simulink library "Kitchen_Lib"  (R2023a)
settings: Solver=VariableStepAuto  StartTime=0.0  StopTime=10.0  RelTol=1e-3  EnableMultiTasking=on
undefined symbols (not defined in the file): Kitc_BusTyp_P, Kitc_BusTypSkyr_C, Kitc_ColrLedColrls_C, Kitc_ColrLedGrn_C, Kitc_ColrLedRed_C, Kitc_ColrLedYlw_C, Kitc_StDgnWtrTank_C, Kitc_StElecPlugScktOffByClmp50_P, Kitc_StsDlyBlink_C, Kitc_StsErrBlink_C, Kitc_StsFctAcvn_P, Kitc_StsInfoBlink_C, Kitc_StsKitchnOffAutoIgOff_P, Kitc_StsKitchnOffBySwt_P, Kitc_StsKitchnOffDoorLockd_P, Kitc_StsKitchnOffIgOff_P, Kitc_StsKitchnOffUv_P, Kitc_StsKitchnOnBySwt_P, Kitc_StsKitchnOnNVM_P, Kitc_StsLedOff_C, Kitc_StsLedOn_C, Kitc_StsLrgCnsAcv_P, Kitc_StTrfrAnSwtInstd_P, Kitc_StTrfrSwtInstd_P, Kitc_TiKitcRefgtrOffDly_P, Kitc_ULowrThdBat_C, Kitc_UUpprThdBat_C, Kitc_ValFalse_C, Kitc_ValPwmFreq2_C, Kitc_ValPwmFreq_C, Kitc_ValTrue_C
libraries: MAN_Library x50, E2E_Lib x3
(part 3 of 13)

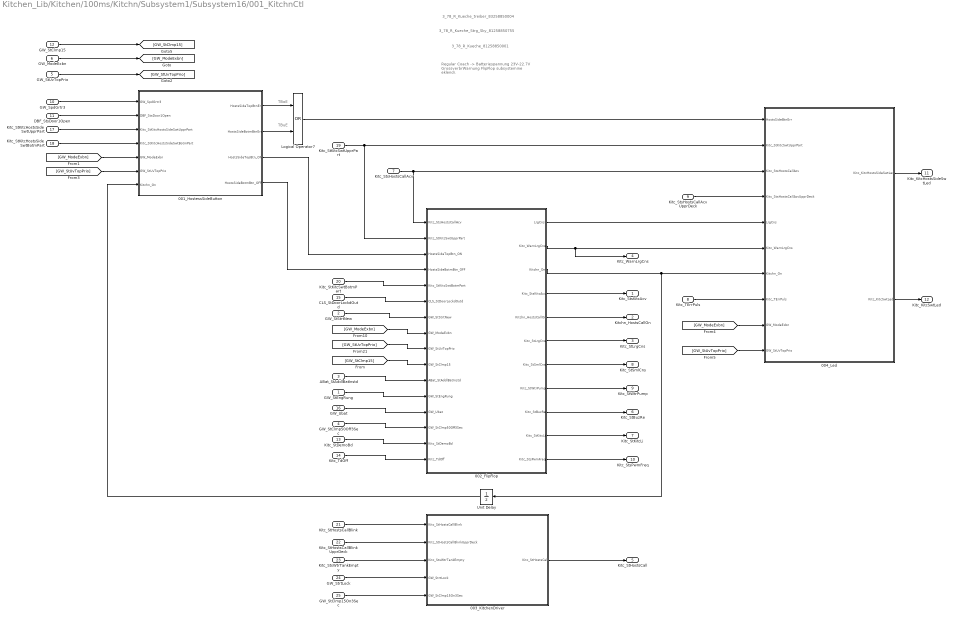
== system Kitchen_Lib/Kitchen/100ms/Kitchn/Subsystem1/Subsystem16/001_KitchnCtl ==
  note: 3_78_R_Kueche_treiber_83258850004
  note: Regular Coach -> Batteriespannung 23V-22.7V
      | GrossverbrWarnung
      |
      | FlipFlop subsystemine eklendi.
  note: 3_78_R_Kueche_81258850001
  note: TBuE
  note: TBoE
  note: 3_78_R_Kueche_Strg_Sky_81258850755
  GW_StEngRung : Inport
  "GW_StStrtNew " : Inport  Port=2
  ABat_StAddlBatInstd : Inport  Port=3
  "GW_StClmp50Off3Sec " : Inport  Port=4
  "GW_StUvTopPrio " : Inport  Port=5
  "GW_ModeExbn " : Inport  Port=6
  Kitc_StsHostsCallAcv : Inport  Port=7
  Kitc_TErrPuls : Inport  Port=8
  Kitc_StsHostsCallAcvUpprDeck : Inport  Port=9
  GW_SpdGrtr3 : Inport  Port=10
  DBF_StsDoor1Open : Inport  Port=11
  GW_StClmp15 : Inport  Port=12
  Kitc_StDemoBd : Inport  Port=13
  Kitc_TdOff : Inport  Port=14
  CLS_StDoorLockdOutd : Inport  Port=15
  "GW_Ubat " : Inport  Port=16
  Kitc_StKitcHostsSideSwtUpprPart : Inport  Port=17
  Kitc_StKitcHostsSideSwtBotmPart : Inport  Port=18
  Kitc_StKitcSwtUpprPart : Inport  Port=19
  Kitc_StKitcSwtBotmPart : Inport  Port=20
  Kitc_StHostsCallBlink : Inport  Port=21
  Kitc_StHostsCallBlinkUpprDeck : Inport  Port=22
  Kitc_StsWtrTankEmpty : Inport  Port=23
  "GW_StrtLock " : Inport  Port=24
  "GW_StClmp15On3Sec " : Inport  Port=25
  001_HostessSideButton : Subsystem
  002_FlipFlop : Subsystem
  003_KitchenDriver : Subsystem
  004_Led : Subsystem
  Logical Operator7 : Logic  Operator=OR  AllPortsSameDT=off  OutDataTypeStr=boolean
  Unit Delay : UnitDelay  SampleTime=-1  HasFrameUpgradeWarning=on
  Kitc_StsKitcAcv : Outport
  Kitchn_HostsCallOn : Outport  Port=2
  Kitc_StLrgCns : Outport  Port=3
  Kitc_WarnLrgCns : Outport  Port=4
  Kitc_StHostsCall : Outport  Port=5
  Kitc_StBuzRe : Outport  Port=6
  Kitc_StKitcLi : Outport  Port=7
  Kitc_StSmlCns : Outport  Port=8
  Kitc_StWtrPump : Outport  Port=9
  Kitc_StsPwmFreq : Outport  Port=10
  Kitc_KitcHostsSideSwtLed : Outport  Port=11
  Kitc_KitcSwtLed : Outport  Port=12
  wires:
  Kitc_StKitcSwtUpprPart/1 -> 002_FlipFlop/2(Kitc_StKitcSwtUpprPart), 004_Led/2(Kitc_StKitcSwtUpprPart)
  "GW_ModeExbn "/1 -> [GW_ModeExbn]
  "GW_StUvTopPrio "/1 -> [GW_StUvTopPrio]
  Kitc_StDemoBd/1 -> 002_FlipFlop/15(Kitc_StDemoBd)
  Kitc_TdOff/1 -> 002_FlipFlop/16(Kitc_TdOff)
  GW_StClmp15/1 -> [GW_StClmp15]
  Kitc_StsHostsCallAcv/1 -> 002_FlipFlop/1(Kitc_StsHostsCallAcv), 004_Led/3(Kitc_StsHostsCallAcv)
  Kitc_StsHostsCallAcvUpprDeck/1 -> 004_Led/4(Kitc_StsHostsCallAcvUpprDeck)
  Logical Operator7/1 -> 004_Led/1(HostsSideBtnErr)
  002_FlipFlop/3(Kitchn_On) -> 004_Led/7(Kitchn_On), Unit Delay/1
  Kitc_StKitcSwtBotmPart/1 -> 002_FlipFlop/5(Kitc_StKitcSwtBotmPart)
  CLS_StDoorLockdOutd/1 -> 002_FlipFlop/6(CLS_StDoorLockdOutd)
  [GW_StUvTopPrio] -> 002_FlipFlop/9("GW_StUvTopPrio ")
  [GW_ModeExbn] -> 002_FlipFlop/8("GW_ModeExbn ")
  "GW_StStrtNew "/1 -> 002_FlipFlop/7("GW_StStrtNew ")
  002_FlipFlop/4(Kitc_StsKitcAcv) -> Kitc_StsKitcAcv/1
  002_FlipFlop/5(Kitchn_HostsCallOn) -> Kitchn_HostsCallOn/1
  002_FlipFlop/6(Kitc_StLrgCns) -> Kitc_StLrgCns/1
  ABat_StAddlBatInstd/1 -> 002_FlipFlop/11(ABat_StAddlBatInstd)
  GW_StEngRung/1 -> 002_FlipFlop/12(GW_StEngRung)
  002_FlipFlop/2(Kitc_WarnLrgCns) -> Kitc_WarnLrgCns/1, 004_Led/6(Kitc_WarnLrgCns)
  "GW_StClmp50Off3Sec "/1 -> 002_FlipFlop/14("GW_StClmp50Off3Sec ")
  "GW_Ubat "/1 -> 002_FlipFlop/13("GW_Ubat ")
  002_FlipFlop/1(LrgCns) -> 004_Led/5(LrgCns)
  GW_SpdGrtr3/1 -> 001_HostessSideButton/1(GW_SpdGrtr3)
  DBF_StsDoor1Open/1 -> 001_HostessSideButton/2(DBF_StsDoor1Open)
  Kitc_StKitcHostsSideSwtUpprPart/1 -> 001_HostessSideButton/3(Kitc_StKitcHostsSideSwtUpprPart)
  Kitc_StKitcHostsSideSwtBotmPart/1 -> 001_HostessSideButton/4(Kitc_StKitcHostsSideSwtBotmPart)
  001_HostessSideButton/1(HostsSideTopBtnErr) -> Logical Operator7/1
  001_HostessSideButton/2(HostsSideBotmBtnErr) -> Logical Operator7/2
  001_HostessSideButton/3(HostsSideTopBtn_ON) -> 002_FlipFlop/3(HostsSideTopBtn_ON)
  001_HostessSideButton/4(HostsSideBotmBtn_OFF) -> 002_FlipFlop/4(HostsSideBotmBtn_OFF)
  Kitc_StsWtrTankEmpty/1 -> 003_KitchenDriver/3(Kitc_StsWtrTankEmpty)
  Kitc_StHostsCallBlink/1 -> 003_KitchenDriver/1(Kitc_StHostsCallBlink)
  "GW_StClmp15On3Sec "/1 -> 003_KitchenDriver/5("GW_StClmp15On3Sec ")
  003_KitchenDriver/1(Kitc_StHostsCall) -> Kitc_StHostsCall/1
  "GW_StrtLock "/1 -> 003_KitchenDriver/4("GW_StrtLock ")
  Kitc_StHostsCallBlinkUpprDeck/1 -> 003_KitchenDriver/2(Kitc_StHostsCallBlinkUpprDeck)
  [GW_ModeExbn] -> 001_HostessSideButton/5("GW_ModeExbn ")
  Unit Delay/1 -> 001_HostessSideButton/7(Kitchn_On)
  Kitc_TErrPuls/1 -> 004_Led/8(Kitc_TErrPuls)
  002_FlipFlop/7(Kitc_StSmlCns) -> Kitc_StSmlCns/1
  002_FlipFlop/8(Kitc_StWtrPump) -> Kitc_StWtrPump/1
  002_FlipFlop/9(Kitc_StBuzRe) -> Kitc_StBuzRe/1
  [GW_StUvTopPrio] -> 001_HostessSideButton/6("GW_StUvTopPrio ")
  [GW_ModeExbn] -> 004_Led/9("GW_ModeExbn ")
  [GW_StUvTopPrio] -> 004_Led/10("GW_StUvTopPrio ")
  002_FlipFlop/10(Kitc_StKitcLi) -> Kitc_StKitcLi/1
  [GW_StClmp15] -> 002_FlipFlop/10(GW_StClmp15)
  002_FlipFlop/11(Kitc_StsPwmFreq) -> Kitc_StsPwmFreq/1
  004_Led/1(Kitc_KitcHostsSideSwtLed) -> Kitc_KitcHostsSideSwtLed/1
  004_Led/2(Kitc_KitcSwtLed) -> Kitc_KitcSwtLed/1

== system Kitchen_Lib/Kitchen/100ms/Kitchn/Subsystem1/Subsystem16/002_ElectPlgSckt ==
  note: O_368_Steckdose_mit_KL50_aus_33258850303
  note: Parameter Kueche_Steckd_Aus_Kl50_P is deleted
  "GW_StrtClmp50 " : Inport
  Constant1 : Constant  Value=Kitc_StElecPlugScktOffByClmp50_P
  Constant2 : Constant  Value=Kitc_ValFalse_C
  Logical Operator : Logic  Operator=NOT  AllPortsSameDT=off  OutDataTypeStr=boolean
  Logical Operator1 : Logic  AllPortsSameDT=off  OutDataTypeStr=boolean
  Multiport Switch : MultiPortSwitch  DataPortOrder=Zero-based contiguous  Inputs=2  zeroidx=on  SaturateOnIntegerOverflow=off  InputSameDT=off
  Kitc_StElecPlgSckt : Outport
  wires:
  Multiport Switch/1 -> Kitc_StElecPlgSckt/1
  Constant2/1 -> Multiport Switch/1
  "GW_StrtClmp50 "/1 -> Logical Operator1/1
  Logical Operator/1 -> Multiport Switch/2
  Logical Operator1/1 -> Multiport Switch/3, Logical Operator/1
  Constant1/1 -> Logical Operator1/2

== system Kitchen_Lib/Kitchen/100ms/Kitchn/Subsystem1/Subsystem16/003_Refgtr ==
  note: O_368_Kuehlschrank_33258850044
  note: 3_78_R_Kuehlschrank_vorne _81258850186
  note: Parameter
      | Kueche_Kuehlbox_nur_bei_KL15_P
      | is deleted
  note: Parameter
      | Kueche_Kuehlbox_nur_bei_Motorlauf_P
      | is deleted
  GW_StClmp15 : Inport
  "GW_StEngAcv " : Inport  Port=2
  GW_StClmpRdo : Inport  Port=3
  "GW_StUvLoPrio " : Inport  Port=4
  "GW_StUvTopPrio " : Inport  Port=5
  Constant : Constant  Value=Kitc_TiKitcRefgtrOffDly_P
  Constant2 : Constant  Value=Kitc_ValFalse_C
  Constant3 : Constant  Value=Kitc_ValFalse_C
  Data Store Read : DataStoreRead  DataStoreName=Kitc_TiKitcRefgtrOffDlyNv  IndexOptions=Index vector (dialog)  Indices=1  OutputSizes=1
  Data Type Conversion : DataTypeConversion  OutDataTypeStr=uint32  SaturateOnIntegerOverflow=off  RndMeth=Floor
  Data Type Conversion1 : DataTypeConversion  OutDataTypeStr=boolean  SaturateOnIntegerOverflow=off  RndMeth=Floor
  Logical Operator{,3,7..8} (4 alike) : Logic  Operator=NOT  AllPortsSameDT=off  OutDataTypeStr=boolean
  Logical Operator{1,4,6,9} (4 alike) : Logic  AllPortsSameDT=off  OutDataTypeStr=boolean
  Logical Operator2 : Logic  Inputs=3  AllPortsSameDT=off  OutDataTypeStr=boolean
  Logical Operator5 : Logic  Operator=OR  Inputs=3  AllPortsSameDT=off  OutDataTypeStr=boolean
  Switch : Switch  Criteria=u2 ~= 0  SaturateOnIntegerOverflow=off  InputSameDT=off
  Terminator4 : Terminator
  TurnOffDelay : MAN_Library/TurnOffDelay  CycleTime=Cycle Time: 10 Ms
  Kitc_StRefgtr : Outport
  "Kitc_StFrntRefgtr " : Outport  Port=2
  wires:
  Data Type Conversion1/1 -> Switch/2
  Constant/1 -> Switch/3
  Data Store Read/1 -> Switch/1, Data Type Conversion1/1
  Switch/1 -> Data Type Conversion/1
  Constant2/1 -> Logical Operator1/2, Logical Operator/1
  Logical Operator/1 -> Logical Operator2/1
  GW_StClmpRdo/1 -> Logical Operator2/2
  Constant3/1 -> Logical Operator4/1, Logical Operator3/1
  Logical Operator3/1 -> Logical Operator2/3
  "GW_StEngAcv "/1 -> Logical Operator4/2
  Logical Operator2/1 -> Logical Operator5/2
  Logical Operator1/1 -> Logical Operator5/1
  Logical Operator4/1 -> Logical Operator5/3
  Logical Operator5/1 -> TurnOffDelay/1
  TurnOffDelay/1 -> Logical Operator6/1
  Logical Operator6/1 -> Kitc_StRefgtr/1
  "GW_StUvLoPrio "/1 -> Logical Operator7/1
  Logical Operator7/1 -> Logical Operator6/2
  "GW_StUvTopPrio "/1 -> Logical Operator8/1
  Logical Operator8/1 -> Logical Operator9/1
  Logical Operator9/1 -> "Kitc_StFrntRefgtr "/1
  GW_StClmp15/1 -> Logical Operator1/1, Logical Operator9/2
  Data Type Conversion/1 -> TurnOffDelay/2
  TurnOffDelay/2 -> Terminator4/1

== system Kitchen_Lib/Kitchen/100ms/Kitchn/Subsystem1/Subsystem16/004_Trfr ==
  note: 3_78_R_Umformer_81258850049
  "Kitc_StTrfrSwt " : Inport
  GW_StClmp15 : Inport  Port=2
  "GW_StUvNormPrio " : Inport  Port=3
  Kitc_StTrfrSwtUpprPart : Inport  Port=4
  Kitc_StTrfrSwtTopBtn : Inport  Port=5
  Kitc_StTrfrSwtLowrPart : Inport  Port=6
  Kitc_StTrfrBotmBtm : Inport  Port=7
  Kitc_StTrfrWoutNewStrt : Inport  Port=8
  "GW_StClmp50Off3Sec " : Inport  Port=9
  ABat_StAddlBatInstd : Inport  Port=10
  "GW_StStrtNew " : Inport  Port=11
  GW_StEngRung : Inport  Port=12
  Kitc_StsKitcAcv : Inport  Port=13
  001_AutomaticControlKitchenRelease : Subsystem
  002_FlipFlop : Subsystem
  003_TrfrSwtLed : Subsystem
  Constant13 : Constant  Value=Kitc_StTrfrSwtInstd_P
  Constant2 : Constant  Value=Kitc_ValTrue_C
  Constant3 : Constant  Value=Kitc_StTrfrAnSwtInstd_P
  Ground : Ground
  Ground1 : Ground
  LEDSignal_Subsytem : E2E_Lib/LEDSignal_Subsytem
  Logical Operator1 : Logic  Operator=OR  Inputs=3  AllPortsSameDT=off  OutDataTypeStr=boolean
  Logical Operator2 : Logic  AllPortsSameDT=off  OutDataTypeStr=boolean
  Logical Operator5 : Logic  Operator=NOT  AllPortsSameDT=off  OutDataTypeStr=boolean
  Multiport Switch : MultiPortSwitch  DataPortOrder=Zero-based contiguous  Inputs=2  zeroidx=on  SaturateOnIntegerOverflow=off  InputSameDT=off
  PushPull : Subsystem
  Kitc_StTrfrInstd : Outport
  Kitc_StTrfrHiSide : Outport  Port=2
  Kitc_StTrfrLoSide : Outport  Port=3
  Kitc_TrfrSwtLed : Outport  Port=4
  wires:
  "Kitc_StTrfrSwt "/1 -> Logical Operator1/1
  Constant13/1 -> Logical Operator1/2
  Multiport Switch/1 -> Logical Operator2/2
  "GW_StClmp50Off3Sec "/1 -> Logical Operator5/1
  Logical Operator2/1 -> PushPull/1(In1)
  PushPull/1(HS) -> Kitc_StTrfrHiSide/1
  PushPull/2(LS) -> Kitc_StTrfrLoSide/1
  Constant2/1 -> Kitc_StTrfrInstd/1
  Logical Operator1/1 -> Multiport Switch/1, 002_FlipFlop/1(TrfrSwt)
  002_FlipFlop/1(Fnc_On) -> Multiport Switch/3, 003_TrfrSwtLed/1(Fnc_On)
  Kitc_StTrfrSwtUpprPart/1 -> 002_FlipFlop/2(Kitc_StTrfrSwtUpprPart)
  Kitc_StTrfrSwtTopBtn/1 -> 002_FlipFlop/3(Kitc_StTrfrSwtTopBtn)
  Kitc_StTrfrSwtLowrPart/1 -> 002_FlipFlop/4(Kitc_StTrfrSwtLowrPart)
  Kitc_StTrfrBotmBtm/1 -> 002_FlipFlop/5(Kitc_StTrfrBotmBtm)
  "GW_StStrtNew "/1 -> 002_FlipFlop/6("GW_StStrtNew ")
  Kitc_StTrfrWoutNewStrt/1 -> 002_FlipFlop/7(Kitc_StTrfrWoutNewStrt)
  [GW_StEngRung] -> 002_FlipFlop/8(GW_StEngRung)
  [ABat_StAddlBatInstd] -> 002_FlipFlop/9(ABat_StAddlBatInstd)
  [GW_StClmp15] -> 002_FlipFlop/10(GW_StClmp15)
  [GW_StUvNormPrio] -> 002_FlipFlop/11("GW_StUvNormPrio ")
  Logical Operator5/1 -> Logical Operator2/1
  GW_StClmp15/1 -> [GW_StClmp15], 001_AutomaticControlKitchenRelease/1(GW_StClmp15)
  "GW_StUvNormPrio "/1 -> [GW_StUvNormPrio], 001_AutomaticControlKitchenRelease/2("GW_StUvNormPrio ")
  ABat_StAddlBatInstd/1 -> [ABat_StAddlBatInstd], 001_AutomaticControlKitchenRelease/3(ABat_StAddlBatInstd)
  GW_StEngRung/1 -> 001_AutomaticControlKitchenRelease/4(GW_StEngRung), [GW_StEngRung]
  Kitc_StsKitcAcv/1 -> 001_AutomaticControlKitchenRelease/5(Kitc_StsKitcAcv)
  001_AutomaticControlKitchenRelease/1(Kitchen) -> Multiport Switch/2
  Constant3/1 -> Logical Operator1/3
  003_TrfrSwtLed/1(Kitc_ColrTrfrSwtLed) -> LEDSignal_Subsytem/1
  003_TrfrSwtLed/2(Kitc_StsTrfrSwtLed) -> LEDSignal_Subsytem/2
  Ground/1 -> LEDSignal_Subsytem/3
  Ground1/1 -> LEDSignal_Subsytem/4
  LEDSignal_Subsytem/1 -> Kitc_TrfrSwtLed/1

== system Kitchen_Lib/Kitchen/100ms/Kitchn/Subsystem1/Subsystem17/UINT32_Signal ==
  UINT32_SignalIn : Inport
  Constant : Constant  Value=uint32(0)
  Constant1 : Constant  Value=uint32(1)
  Constant2 : Constant  Value=uint32(4294967294)
  Constant3 : Constant  Value=uint32(4294967295)
  Data Type Conversion : DataTypeConversion  OutDataTypeStr=uint32  SaturateOnIntegerOverflow=off  RndMeth=Floor
  Relational Operator{,1..3} (4 alike) : RelationalOperator  Operator===  OutDataTypeStr=boolean  InputSameDT=off
  Terminator : Terminator
  Terminator1 : Terminator
  Error : Outport
  NotInstalled_NotAvailable : Outport  Port=2
  wires:
  Relational Operator3/1 -> NotInstalled_NotAvailable/1
  Relational Operator2/1 -> Error/1
  Data Type Conversion/1 -> Relational Operator/1, Relational Operator1/1, Relational Operator2/1, Relational Operator3/1
  Constant/1 -> Relational Operator/2
  UINT32_SignalIn/1 -> Data Type Conversion/1
  Constant3/1 -> Relational Operator3/2
  Constant1/1 -> Relational Operator1/2
  Relational Operator/1 -> Terminator/1
  Relational Operator1/1 -> Terminator1/1
  Constant2/1 -> Relational Operator2/2

== system Kitchen_Lib/Kitchen/100ms/Kitchn/Subsystem1/Subsystem19/003_TrfrSwtLed ==
  Fnc_On : Inport
  Constant12 : Constant  Value=Kitc_ColrLedColrls_C
  Constant13 : Constant  Value=Kitc_ColrLedYlw_C
  Constant4 : Constant  Value=Kitc_StsLedOff_C
  Constant5 : Constant  Value=Kitc_StsLedOn_C
  Ground : Ground
  Ground1 : Ground
  LEDSignal_Subsytem : Subsystem  AncestorBlock=E2E_Lib/LEDSignal_Subsytem
  Multiport Switch1 : MultiPortSwitch  DataPortOrder=Zero-based contiguous  Inputs=2  zeroidx=on  SaturateOnIntegerOverflow=off  InputSameDT=off
  Multiport Switch2 : MultiPortSwitch  DataPortOrder=Zero-based contiguous  Inputs=2  zeroidx=on  SaturateOnIntegerOverflow=off  InputSameDT=off
  Kitc_TrfrSwtLed : Outport
  wires:
  LEDSignal_Subsytem/1(Led) -> Kitc_TrfrSwtLed/1
  Ground/1 -> LEDSignal_Subsytem/3(Error)
  Ground1/1 -> LEDSignal_Subsytem/4(NA)
  Multiport Switch2/1 -> LEDSignal_Subsytem/2(Status)
  Multiport Switch1/1 -> LEDSignal_Subsytem/1(Color)
  Constant5/1 -> Multiport Switch2/3
  Constant4/1 -> Multiport Switch2/2
  Constant12/1 -> Multiport Switch1/2
  Constant13/1 -> Multiport Switch1/3
  Fnc_On/1 -> Multiport Switch1/1, Multiport Switch2/1

== system Kitchen_Lib/Kitchen/100ms/Kitchn/Subsystem1/Subsystem19/BusTypeSelection ==
  GW_BusTyp : Inport
  Constant : Constant  Value=uint8(0)
  Constant1 : Constant  Value=uint8(1)
  Constant2 : Constant  Value=uint8(2)
  Constant3 : Constant  Value=uint8(3)
  Constant4 : Constant  Value=uint8(4)
  Constant5 : Constant  Value=uint8(5)
  Constant6 : Constant  Value=uint8(6)
  Relational Operator{,1..6} (7 alike) : RelationalOperator  Operator===  OutDataTypeStr=boolean  InputSameDT=off
  Terminator : Terminator
  BusTypCityStep1 : Outport
  BusTypCityStep2 : Outport  Port=2
  BusTypCoach : Outport  Port=3
  BusTypIntercity : Outport  Port=4
  BusTypSky : Outport  Port=5
  BusTypElec : Outport  Port=6
  wires:
  Constant2/1 -> Relational Operator1/2
  Constant3/1 -> Relational Operator2/2
  Relational Operator2/1 -> BusTypCoach/1
  Relational Operator1/1 -> BusTypCityStep2/1
  Relational Operator3/1 -> BusTypIntercity/1
  Relational Operator/1 -> BusTypCityStep1/1
  Constant1/1 -> Relational Operator/2
  Constant4/1 -> Relational Operator3/2
  Constant/1 -> Relational Operator4/2
  Relational Operator4/1 -> Terminator/1
  Relational Operator5/1 -> BusTypSky/1
  Constant5/1 -> Relational Operator5/2
  Constant6/1 -> Relational Operator6/2
  GW_BusTyp/1 -> Relational Operator4/1, Relational Operator6/1, Relational Operator5/1, Relational Operator3/1, Relational Operator2/1, Relational Operator1/1, Relational Operator/1
  Relational Operator6/1 -> BusTypElec/1

== system Kitchen_Lib/Kitchen/100ms/Kitchn/Subsystem1/Subsystem19/Cluster_Message ==
  GW_StUvTopPrio : Inport
  Kitc_KitchenReleased : Inport  Port=2
  Ground : Ground
  Logical Operator : Logic  AllPortsSameDT=off  OutDataTypeStr=boolean
  Subsystem2 : Subsystem  Commented=on
  Kitc_KtchnLowBttryNotRlsd : Outport
  Kitch_dispKitchenPssngrReqAcv : Outport  Port=2
  wires:
  Ground/1 -> Kitch_dispKitchenPssngrReqAcv/1
  Logical Operator/1 -> Kitc_KtchnLowBttryNotRlsd/1
  Kitc_KitchenReleased/1 -> Logical Operator/2
  GW_StUvTopPrio/1 -> Logical Operator/1

== system Kitchen_Lib/Kitchen/100ms/Kitchn/Subsystem1/Subsystem19/FallingEdgeDetection ==
  CLK : Inport
  Constant : Constant  Value=boolean(0)  OutDataTypeStr=boolean
  Data Type Conversion1 : DataTypeConversion  OutDataTypeStr=boolean  SaturateOnIntegerOverflow=off  RndMeth=Floor
  Logical Operator1 : Logic  AllPortsSameDT=off  OutDataTypeStr=boolean
  Relational Operator2 : RelationalOperator  Operator=~=  OutDataTypeStr=boolean  InputSameDT=off
  Relational Operator3 : RelationalOperator  Operator===  OutDataTypeStr=boolean  InputSameDT=off
  Unit Delay1 : UnitDelay  SampleTime=-1  HasFrameUpgradeWarning=on
  Q : Outport
  wires:
  Unit Delay1/1 -> Relational Operator2/1
  Relational Operator2/1 -> Logical Operator1/1
  Relational Operator3/1 -> Logical Operator1/2
  Logical Operator1/1 -> Q/1
  CLK/1 -> Data Type Conversion1/1
  Constant/1 -> Relational Operator3/2
  Data Type Conversion1/1 -> Relational Operator3/1, Relational Operator2/2, Unit Delay1/1

== system Kitchen_Lib/Kitchen/100ms/Kitchn/Subsystem1/Subsystem19/KSW_Battery ==
  Kitchn_On : Inport
  "GW_Ubat " : Inport  Port=2
  GW_StClmp15 : Inport  Port=3
  "GW_StUvTopPrio " : Inport  Port=4
  "GW_ModeExbn " : Inport  Port=5
  "GW_StClmp50Off3Sec " : Inport  Port=6
  CLS_StDoorLockdOutd : Inport  Port=7
  Kitc_StsHostsCallAcv : Inport  Port=8
  GW_StEngRung : Inport  Port=9
  ABat_StAddlBatInstd : Inport  Port=10
  BatteryVoltageUnder22700mV : Subsystem
  BatteryVoltageUnder23V : Subsystem
  KitchenActivation : Subsystem
  Logical Operator51 : Logic  Operator=OR  AllPortsSameDT=off  OutDataTypeStr=boolean
  Kitc_StBuzRe : Outport
  Kitc_WarnLrgCns : Outport  Port=2
  wires:
  Logical Operator51/1 -> BatteryVoltageUnder23V/2(EngOrAddlBat), KitchenActivation/9(EngOrAddlBat), BatteryVoltageUnder22700mV/2(EngOrAddlBat)
  "GW_Ubat "/1 -> BatteryVoltageUnder23V/1(GW_Ubat), BatteryVoltageUnder22700mV/3("GW_Ubat ")
  BatteryVoltageUnder22700mV/1(BatUUnder22700mV) -> KitchenActivation/5(BatUUnder22.7V)
  BatteryVoltageUnder23V/2(Kitc_WarnLrgCns) -> Kitc_WarnLrgCns/1
  BatteryVoltageUnder23V/3(Kitc_StBuzRe) -> Kitc_StBuzRe/1
  BatteryVoltageUnder23V/1(LrgCnsOff) -> KitchenActivation/6(LrgCnsOff)
  Kitchn_On/1 -> BatteryVoltageUnder22700mV/1(Kitchn_On), [Kitchn_On]
  [Kitchn_On] -> BatteryVoltageUnder23V/3(Kitchn_On)
  Kitc_StsHostsCallAcv/1 -> BatteryVoltageUnder23V/4(Kitc_StsHostsCallAcv)
  "GW_StClmp50Off3Sec "/1 -> KitchenActivation/1("GW_StClmp50Off3Sec ")
  "GW_StUvTopPrio "/1 -> KitchenActivation/2("GW_StUvTopPrio ")
  "GW_ModeExbn "/1 -> KitchenActivation/3("GW_ModeExbn ")
  CLS_StDoorLockdOutd/1 -> KitchenActivation/4(CLS_StDoorLockdOutd)
  GW_StClmp15/1 -> KitchenActivation/8(GW_StClmp15)
  [Kitchn_On] -> KitchenActivation/7(Kitchn_On)
  ABat_StAddlBatInstd/1 -> Logical Operator51/1
  GW_StEngRung/1 -> Logical Operator51/2

== system Kitchen_Lib/Kitchen/100ms/Kitchn/Subsystem1/Subsystem19/KitchenActive ==
  Kitchn_On : Inport
  GW_StClmp15 : Inport  Port=2
  ABat_StAddlBatInstd : Inport  Port=3
  GW_StEngRung : Inport  Port=4
  Kitc_BusTypSkyr : Inport  Port=5
  Logical Operator50 : Logic  Inputs=3  AllPortsSameDT=off  OutDataTypeStr=boolean
  Logical Operator51 : Logic  Operator=OR  AllPortsSameDT=off  OutDataTypeStr=boolean
  Multiport Switch : MultiPortSwitch  DataPortOrder=Zero-based contiguous  Inputs=2  zeroidx=on  SaturateOnIntegerOverflow=off  InputSameDT=off
  Kitc_StsKitcAcv : Outport
  wires:
  Kitc_BusTypSkyr/1 -> Multiport Switch/1
  Kitchn_On/1 -> Multiport Switch/2, Logical Operator50/2
  GW_StEngRung/1 -> Logical Operator51/2
  ABat_StAddlBatInstd/1 -> Logical Operator51/1
  Logical Operator51/1 -> Logical Operator50/3
  Logical Operator50/1 -> Multiport Switch/3
  Multiport Switch/1 -> Kitc_StsKitcAcv/1
  GW_StClmp15/1 -> Logical Operator50/1

== system Kitchen_Lib/Kitchen/100ms/Kitchn/Subsystem1/Subsystem19/KitchenDriver ==
  note: 3_78_R_Kueche_treiber_83258850004
  Kitc_StHostsCallBlink : Inport
  Kitc_StHostsCallBlinkUpprDeck : Inport  Port=2
  Constant : Constant  Value=uint16(400)
  Data Type Conversion : DataTypeConversion  OutDataTypeStr=uint16  SaturateOnIntegerOverflow=off  RndMeth=Floor
  Data Type Conversion1 : DataTypeConversion  OutDataTypeStr=uint16  SaturateOnIntegerOverflow=off  RndMeth=Floor
  Logical Operator1 : Logic  Operator=OR  AllPortsSameDT=off  OutDataTypeStr=boolean
  Kitc_StHostsCall : Outport
  Kitc_PwmHostsCall : Outport  Port=2
  wires:
  Data Type Conversion1/1 -> Kitc_StHostsCall/1
  Data Type Conversion/1 -> Kitc_PwmHostsCall/1
  Constant/1 -> Data Type Conversion/1
  Logical Operator1/1 -> Data Type Conversion1/1
  Kitc_StHostsCallBlink/1 -> Logical Operator1/1
  Kitc_StHostsCallBlinkUpprDeck/1 -> Logical Operator1/2

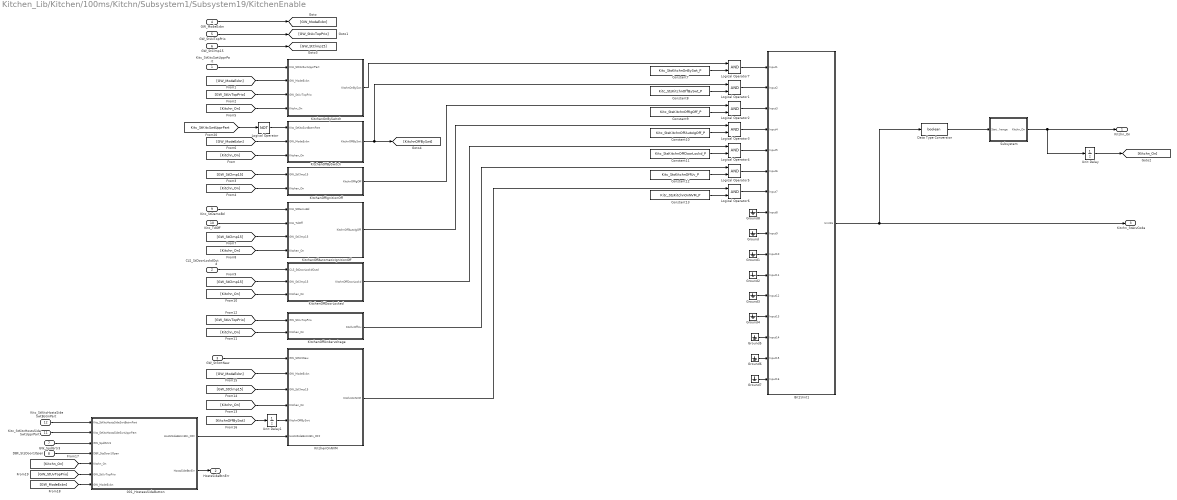
== system Kitchen_Lib/Kitchen/100ms/Kitchn/Subsystem1/Subsystem19/KitchenEnable ==
  Kitc_StKitcSwtUpprPart : Inport
  CLS_StDoorLockdOutd : Inport  Port=2
  "GW_StStrtNew " : Inport  Port=3
  "GW_ModeExbn " : Inport  Port=4
  "GW_StUvTopPrio " : Inport  Port=5
  GW_StClmp15 : Inport  Port=6
  GW_SpdGrtr3 : Inport  Port=7
  DBF_StsDoor1Open : Inport  Port=8
  Kitc_StDemoBd : Inport  Port=9
  Kitc_TdOff : Inport  Port=10
  Kitc_StKitcHostsSideSwtUpprPart : Inport  Port=11
  Kitc_StKitcHostsSideSwtBotmPart : Inport  Port=12
  001_HostessSideButton : Subsystem
  Bit2Uint1 : Subsystem  AncestorBlock=MAN_Library/Bit2Uint1
  Constant10 : Constant  Value=Kitc_StsKitchnOffAutoIgOff_P
  Constant11 : Constant  Value=Kitc_StsKitchnOffDoorLockd_P
  Constant12 : Constant  Value=Kitc_StsKitchnOffUv_P
  Constant13 : Constant  Value=Kitc_StsKitchnOnNVM_P
  Constant7 : Constant  Value=Kitc_StsKitchnOnBySwt_P
  Constant8 : Constant  Value=Kitc_StsKitchnOffBySwt_P
  Constant9 : Constant  Value=Kitc_StsKitchnOffIgOff_P
  Data Type Conversion : DataTypeConversion  OutDataTypeStr=boolean  SaturateOnIntegerOverflow=off  RndMeth=Floor
  Ground{,1..8} (9 alike) : Ground
  KitchenOffAutomaticIgnitionOff : Subsystem
  KitchenOffBySwitch : Subsystem
  KitchenOffDoorLocked : Subsystem
  KitchenOffIgnitionOff : Subsystem
  KitchenOffUndervoltage : Subsystem
  KitchenOnBySwitch : Subsystem
  KitchenOnNVM : Subsystem
  Logical Operator : Logic  Operator=NOT  AllPortsSameDT=off  OutDataTypeStr=boolean
  Logical Operator{1..7} (7 alike) : Logic  AllPortsSameDT=off  OutDataTypeStr=boolean
  Subsystem : Subsystem
  Unit Delay : UnitDelay  SampleTime=-1  HasFrameUpgradeWarning=on
  Unit Delay1 : UnitDelay  SampleTime=-1  HasFrameUpgradeWarning=on
  Kitchn_On : Outport
  HostsSideBtnErr : Outport  Port=2
  Kitchn_StAcvCode : Outport  Port=3
  wires:
  Logical Operator/1 -> KitchenOffBySwitch/1(Kitc_StKitcSwtBotmPart)
  Constant13/1 -> Logical Operator6/2
  Constant12/1 -> Logical Operator5/2
  Constant11/1 -> Logical Operator4/2
  Constant10/1 -> Logical Operator3/2
  Constant9/1 -> Logical Operator2/2
  Constant7/1 -> Logical Operator7/2
  Kitc_StKitcHostsSideSwtBotmPart/1 -> 001_HostessSideButton/1(Kitc_StKitcHostsSideSwtBotmPart)
  Kitc_StKitcHostsSideSwtUpprPart/1 -> 001_HostessSideButton/2(Kitc_StKitcHostsSideSwtUpprPart)
  KitchenOnNVM/1("KitchnOnNVM  ") -> Logical Operator6/1
  Logical Operator6/1 -> Bit2Uint1/7(Input7)
  KitchenOffUndervoltage/1(KitchnOffUv) -> Logical Operator5/1
  Logical Operator5/1 -> Bit2Uint1/6(Input6)
  KitchenOffDoorLocked/1(KitchnOffDoorLockd) -> Logical Operator4/1
  Logical Operator4/1 -> Bit2Uint1/5(Input5)
  KitchenOffAutomaticIgnitionOff/1("KitchnOffAutoIgOff ") -> Logical Operator3/1
  Logical Operator3/1 -> Bit2Uint1/4(Input4)
  Logical Operator2/1 -> Bit2Uint1/3(Input3)
  KitchenOffIgnitionOff/1(KitchnOffIgOff) -> Logical Operator2/1
  Logical Operator1/1 -> Bit2Uint1/2(Input2)
  Constant8/1 -> Logical Operator1/2
  Logical Operator7/1 -> Bit2Uint1/1(Input1)
  KitchenOnBySwitch/1("KitchnOnBySwt ") -> Logical Operator7/1
  Ground8/1 -> Bit2Uint1/8(Input8)
  001_HostessSideButton/1(HostsSideBotmBtn_OFF) -> KitchenOnNVM/6(HostsSideBotmBtn_OFF)
  Ground7/1 -> Bit2Uint1/16(Input16)
  Ground6/1 -> Bit2Uint1/15(Input15)
  Ground5/1 -> Bit2Uint1/14(Input14)
  Ground4/1 -> Bit2Uint1/13(Input13)
  Ground3/1 -> Bit2Uint1/12(Input12)
  Ground2/1 -> Bit2Uint1/11(Input11)
  Ground1/1 -> Bit2Uint1/10(Input10)
  Ground/1 -> Bit2Uint1/9(Input9)
  Bit2Uint1/1(Uint16) -> Kitchn_StAcvCode/1, Data Type Conversion/1
  DBF_StsDoor1Open/1 -> 001_HostessSideButton/4(DBF_StsDoor1Open)
  GW_SpdGrtr3/1 -> 001_HostessSideButton/3(GW_SpdGrtr3)
  [Kitchn_On] -> 001_HostessSideButton/5(Kitchn_On)
  [GW_StUvTopPrio] -> 001_HostessSideButton/6("GW_StUvTopPrio ")
  [GW_ModeExbn] -> 001_HostessSideButton/7("GW_ModeExbn ")
  001_HostessSideButton/2(HostsSideBtnErr) -> HostsSideBtnErr/1
  Subsystem/1(Kitchn_On) -> Unit Delay/1, Kitchn_On/1
  Data Type Conversion/1 -> Subsystem/1(StateChange)
  "GW_ModeExbn "/1 -> [GW_ModeExbn]
  "GW_StUvTopPrio "/1 -> [GW_StUvTopPrio]
  GW_StClmp15/1 -> [GW_StClmp15]
  Unit Delay/1 -> [Kitchn_On]
  Kitc_StKitcSwtUpprPart/1 -> KitchenOnBySwitch/1(Kitc_StKitcSwtUpprPart)
  [Kitc_StKitcSwtUpprPart] -> Logical Operator/1
  KitchenOffBySwitch/1(KitchnOffBySwt) -> Logical Operator1/1, [KitchnOffBySwt]
  Kitc_StDemoBd/1 -> KitchenOffAutomaticIgnitionOff/1(Kitc_StDemoBd)
  Kitc_TdOff/1 -> KitchenOffAutomaticIgnitionOff/2(Kitc_TdOff)
  CLS_StDoorLockdOutd/1 -> KitchenOffDoorLocked/1(CLS_StDoorLockdOutd)
  "GW_StStrtNew "/1 -> KitchenOnNVM/1("GW_StStrtNew ")
  [Kitchn_On] -> KitchenOnBySwitch/4(Kitchn_On)
  [GW_ModeExbn] -> KitchenOnBySwitch/2("GW_ModeExbn ")
  [GW_StUvTopPrio] -> KitchenOnBySwitch/3("GW_StUvTopPrio ")
  [GW_StClmp15] -> KitchenOffIgnitionOff/1(GW_StClmp15)
  [Kitchn_On] -> KitchenOffIgnitionOff/2(Kitchen_On)
  [Kitchn_On] -> KitchenOffBySwitch/3(Kitchen_On)
  [GW_ModeExbn] -> KitchenOffBySwitch/2("GW_ModeExbn ")
  [GW_StClmp15] -> KitchenOffAutomaticIgnitionOff/3(GW_StClmp15)
  [Kitchn_On] -> KitchenOffAutomaticIgnitionOff/4(Kitchen_On)
  [GW_StClmp15] -> KitchenOffDoorLocked/2(GW_StClmp15)
  [Kitchn_On] -> KitchenOffDoorLocked/3(Kitchen_On)
  [Kitchn_On] -> KitchenOffUndervoltage/2(Kitchen_On)
  [GW_StUvTopPrio] -> KitchenOffUndervoltage/1("GW_StUvTopPrio ")
  [GW_StClmp15] -> KitchenOnNVM/3(GW_StClmp15)
  [Kitchn_On] -> KitchenOnNVM/4(Kitchen_On)
  [GW_ModeExbn] -> KitchenOnNVM/2("GW_ModeExbn ")
  [KitchnOffBySwt] -> Unit Delay1/1
  Unit Delay1/1 -> KitchenOnNVM/5(KitchnOffBySwt)

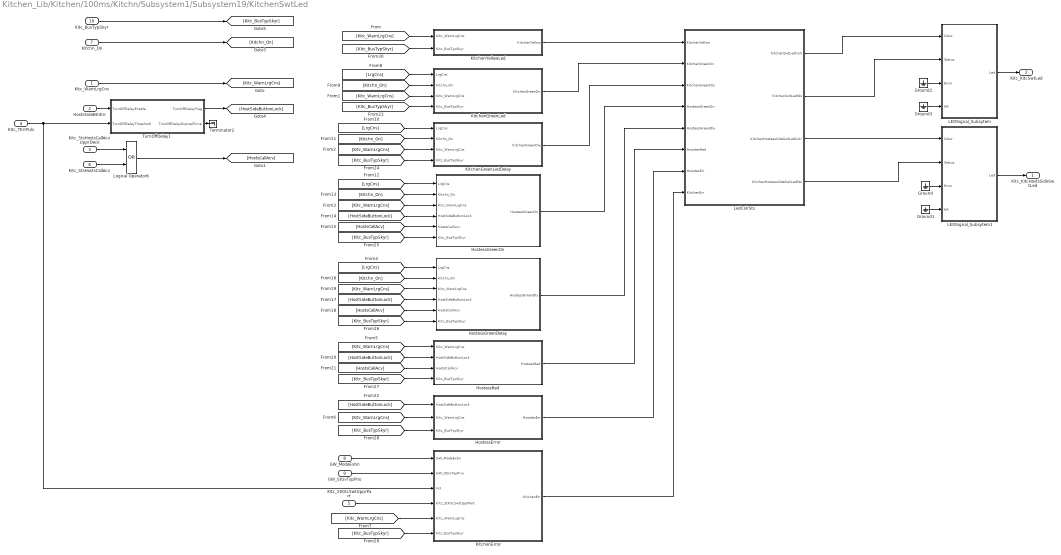
== system Kitchen_Lib/Kitchen/100ms/Kitchn/Subsystem1/Subsystem19/KitchenSwtLed ==
  Kitc_WarnLrgCns : Inport
  HostsSideBtnErr : Inport  Port=2
  Kitc_StsHostsCallAcvUpprDeck : Inport  Port=3
  Kitc_TErrPuls : Inport  Port=4
  Kitc_StKitcSwtUpprPart : Inport  Port=5
  Kitc_StsHostsCallAcv : Inport  Port=6
  Kitchn_On : Inport  Port=7
  "GW_ModeExbn " : Inport  Port=8
  "GW_StUvTopPrio " : Inport  Port=9
  Kitc_BusTypSkyr : Inport  Port=10
  Ground{,1..3} (4 alike) : Ground
  HostessError : Subsystem
  HostessGreenDelay : Subsystem
  HostessGreenOn : Subsystem
  HostessRed : Subsystem
  KitchenError : Subsystem
  KitchenGreenLed : Subsystem
  KitchenGreenLedDelay : Subsystem
  KitchenYellowLed : Subsystem
  LEDSignal_Subsytem : Subsystem  AncestorBlock=E2E_Lib/LEDSignal_Subsytem
  LEDSignal_Subsytem1 : Subsystem  AncestorBlock=E2E_Lib/LEDSignal_Subsytem
  LedColrSts : Subsystem
  Logical Operator6 : Logic  Operator=OR  AllPortsSameDT=off  OutDataTypeStr=boolean
  Terminator2 : Terminator
  TurnOffDelay1 : Subsystem  AncestorBlock=MAN_Library/TurnOffDelay  mask(Turn Off Delay){CycleTime=Cycle Time: 10 Ms}
      mask prompts: CycleTime "Select the Cycle Time:"
      mask help:
      | This is an EDGE DELAY where the turning-off edge is delayed. The delay period is entered at input PT. The output Q is reset after turning off input IN, only after the delay period is over. Output ET counts the time - beginning with the occurrence of the negative edge - until the value set at PT has been reached. The output ET shows the expired time since turning input IN off until the input state of IN is put through to output Q.
      |
      | IN : Timer starting bit
      | PT : Preset time of timer
      | Q  : Time pulse flag
      | ET : Current value of timer
      mask TypeOptions CycleTime: Cycle Time: 1 Ms | Cycle Time: 10 Ms | Cycle Time: 100 Ms | Cycle Time: 1000 Ms
      mask Display:
      | disp('{\bf\fontsize{18}Turn Off Delay}', 'texmode','on');
      | 
      | port_label('input', 1,'IN');
      | port_label('input', 2,'PT');
      | port_label('output',1,'Q');
      | port_label('output',2,'ET');
  Kitc_KitcHostsSideSwtLed : Outport
  Kitc_KitcSwtLed : Outport  Port=2
  wires:
  [Kitc_BusTypSkyr] -> KitchenYellowLed/2(Kitc_BusTypSkyr)
  [Kitc_BusTypSkyr] -> KitchenError/6(Kitc_BusTypSkyr)
  [Kitc_BusTypSkyr] -> HostessError/3(Kitc_BusTypSkyr)
  [Kitc_BusTypSkyr] -> HostessRed/4(Kitc_BusTypSkyr)
  [Kitc_BusTypSkyr] -> HostessGreenDelay/6(Kitc_BusTypSkyr)
  [Kitc_BusTypSkyr] -> HostessGreenOn/6(Kitc_BusTypSkyr)
  [Kitc_BusTypSkyr] -> KitchenGreenLedDelay/4(Kitc_BusTypSkyr)
  [Kitc_BusTypSkyr] -> KitchenGreenLed/4(Kitc_BusTypSkyr)
  Kitc_BusTypSkyr/1 -> [Kitc_BusTypSkyr]
  LedColrSts/1(KitchenSwtLedColr) -> LEDSignal_Subsytem/1(Color)
  LedColrSts/2(KitchenSwtLedSts) -> LEDSignal_Subsytem/2(Status)
  Kitc_WarnLrgCns/1 -> [Kitc_WarnLrgCns]
  KitchenYellowLed/1(KitchenYellow) -> LedColrSts/1(KitchenYellow)
  KitchenGreenLed/1(KitchenGreenOn) -> LedColrSts/2(KitchenGreenOn)
  KitchenGreenLedDelay/1(KitchenGreenDly) -> LedColrSts/3(KitchenGreenDly)
  HostessGreenOn/1(HostessGreenOn) -> LedColrSts/4(HostessGreenOn)
  HostessGreenDelay/1(HostessGreenDly) -> LedColrSts/5(HostessGreenDly)
  HostessRed/1(HostessRed) -> LedColrSts/6(HosstesRed)
  HostessError/1(HosstesErr) -> LedColrSts/7(HosstesErr)
  "GW_ModeExbn "/1 -> KitchenError/1("GW_ModeExbn ")
  "GW_StUvTopPrio "/1 -> KitchenError/2("GW_StUvTopPrio ")
  Kitc_StKitcSwtUpprPart/1 -> KitchenError/4(Kitc_StKitcSwtUpprPart)
  KitchenError/1(KitchenErr) -> LedColrSts/8(KitchenErr)
  TurnOffDelay1/1(TurnOffDelayFlag) -> [HostSideButtonLock]
  TurnOffDelay1/2(TurnOffDelayExpiredTime) -> Terminator2/1
  HostsSideBtnErr/1 -> TurnOffDelay1/1(TurnOffDelayEnable)
  Kitc_StsHostsCallAcv/1 -> Logical Operator6/2
  Kitc_StsHostsCallAcvUpprDeck/1 -> Logical Operator6/1
  Kitc_TErrPuls/1 -> KitchenError/3(In3), TurnOffDelay1/2(TurnOffDelayThreshold)
  Logical Operator6/1 -> [HostsCallAcv]
  Kitchn_On/1 -> [Kitchn_On]
  [Kitc_WarnLrgCns] -> KitchenYellowLed/1(Kitc_WarnLrgCns)
  [Kitc_WarnLrgCns] -> KitchenGreenLed/3(Kitc_WarnLrgCns)
  [Kitc_WarnLrgCns] -> KitchenGreenLedDelay/3(Kitc_WarnLrgCns)
  [Kitc_WarnLrgCns] -> HostessGreenOn/3(Kitc_WarnLrgCns)
  [Kitc_WarnLrgCns] -> HostessRed/1(Kitc_WarnLrgCns)
  [Kitc_WarnLrgCns] -> HostessError/2(Kitc_WarnLrgCns)
  [Kitc_WarnLrgCns] -> KitchenError/5(Kitc_WarnLrgCns)
  [LrgCns] -> KitchenGreenLed/1(LrgCns)
  [Kitchn_On] -> KitchenGreenLed/2(Kitchn_On)
  [Kitchn_On] -> KitchenGreenLedDelay/2(Kitchn_On)
  [LrgCns] -> KitchenGreenLedDelay/1(LrgCns)
  [Kitchn_On] -> HostessGreenOn/2(Kitchn_On)
  [LrgCns] -> HostessGreenOn/1(LrgCns)
  [HostSideButtonLock] -> HostessGreenOn/4(HostSideButtonLock)
  [HostsCallAcv] -> HostessGreenOn/5(HostsCallAcv)
  [Kitc_WarnLrgCns] -> HostessGreenDelay/3(Kitc_WarnLrgCns)
  [LrgCns] -> HostessGreenDelay/1(LrgCns)
  [Kitchn_On] -> HostessGreenDelay/2(Kitchn_On)
  [HostSideButtonLock] -> HostessGreenDelay/4(HostSideButtonLock)
  [HostsCallAcv] -> HostessGreenDelay/5(HostsCallAcv)
  [HostSideButtonLock] -> HostessRed/2(HostSideButtonLock)
  [HostsCallAcv] -> HostessRed/3(HostsCallAcv)
  [HostSideButtonLock] -> HostessError/1(HostSideButtonLock)
  Ground/1 -> LEDSignal_Subsytem1/3(Error)
  Ground1/1 -> LEDSignal_Subsytem1/4(NA)
  LEDSignal_Subsytem1/1(Led) -> Kitc_KitcHostsSideSwtLed/1
  LedColrSts/3(KitchenHostessSideSwtLedColr) -> LEDSignal_Subsytem1/1(Color)
  LedColrSts/4(KitchenHostessSideSwtLedSts) -> LEDSignal_Subsytem1/2(Status)
  LEDSignal_Subsytem/1(Led) -> Kitc_KitcSwtLed/1
  Ground2/1 -> LEDSignal_Subsytem/3(Error)
  Ground3/1 -> LEDSignal_Subsytem/4(NA)

== system Kitchen_Lib/Kitchen/100ms/Kitchn/Subsystem1/Subsystem19/PWMOutput ==
  GW_StClmp15 : Inport
  KitchnOn : Inport  Port=2
  Constant1 : Constant  Value=Kitc_ValPwmFreq2_C
  Constant4 : Constant  Value=Kitc_ValPwmFreq_C
  Data Type Conversion : DataTypeConversion  OutDataTypeStr=boolean  SaturateOnIntegerOverflow=off  RndMeth=Floor
  Gain : Gain  Gain=100  OutDataTypeStr=uint16
  Gain1 : Gain  Gain=100  OutDataTypeStr=uint16
  Logical Operator : Logic  Operator=OR  Inputs=3  AllPortsSameDT=off  OutDataTypeStr=boolean
  Logical Operator1 : Logic  Operator=NOT  AllPortsSameDT=off  OutDataTypeStr=boolean
  Logical Operator50 : Logic  AllPortsSameDT=off  OutDataTypeStr=boolean
  Kitc_StLrgCns : Outport
  Kitc_StSmlCns : Outport  Port=2
  Kitc_StsPwmFreq : Outport  Port=3
  Kitc_StsPwmFreq2 : Outport  Port=4
  Kitc_AcvSkyliner : Outport  Port=5
  Kitc_KitchenReleased : Outport  Port=6
  Kitc_KitchenNotReleased : Outport  Port=7
  wires:
  Logical Operator1/1 -> Kitc_KitchenNotReleased/1
  Logical Operator/1 -> Logical Operator1/1, Kitc_KitchenReleased/1
  [Kitc_StLrgCns] -> Logical Operator/3
  [Kitc_AcvSkyliner] -> Logical Operator/2
  [Kitc_StSmlCns] -> Logical Operator/1
  Data Type Conversion/1 -> Kitc_AcvSkyliner/1, [Kitc_AcvSkyliner]
  Constant1/1 -> Kitc_StsPwmFreq2/1
  Logical Operator50/1 -> Gain/1, Data Type Conversion/1
  GW_StClmp15/1 -> Logical Operator50/1
  KitchnOn/1 -> Gain1/1, Logical Operator50/2
  Gain/1 -> Kitc_StLrgCns/1, [Kitc_StLrgCns]
  Gain1/1 -> Kitc_StSmlCns/1, [Kitc_StSmlCns]
  Constant4/1 -> Kitc_StsPwmFreq/1

== system Kitchen_Lib/Kitchen/100ms/Kitchn/Subsystem1/Subsystem19/Refgtr ==
  note: Parameter
      | Kueche_Kuehlbox_nur_bei_Motorlauf_P
      | is deleted
  note: Parameter
      | Kueche_Kuehlbox_nur_bei_KL15_P
      | is deleted
  note: 3_78_R_Kuehlschrank_vorne _81258850186
  note: O_368_Kuehlschrank_33258850044
  GW_StClmp15 : Inport
  "GW_StUvTopPrio " : Inport  Port=2
  "GW_StEngAcv " : Inport  Port=3
  GW_StClmpRdo : Inport  Port=4
  "GW_StUvLoPrio " : Inport  Port=5
  Toi_ToiInstlldInfo : Inport  Port=6
  Constant : Constant  Value=Kitc_TiKitcRefgtrOffDly_P
  Constant2 : Constant  Value=Kitc_ValFalse_C
  Constant3 : Constant  Value=Kitc_ValFalse_C
  Data Store Read : DataStoreRead  DataStoreName=Kitc_TiKitcRefgtrOffDlyNv  IndexOptions=Index vector (dialog)  Indices=1  OutputSizes=1
  Data Type Conversion : DataTypeConversion  OutDataTypeStr=uint32  SaturateOnIntegerOverflow=off  RndMeth=Floor
  Data Type Conversion1 : DataTypeConversion  OutDataTypeStr=boolean  SaturateOnIntegerOverflow=off  RndMeth=Floor
  Logical Operator{,3,7..8} (4 alike) : Logic  Operator=NOT  AllPortsSameDT=off  OutDataTypeStr=boolean
  Logical Operator{1,4,6,9..10} (5 alike) : Logic  AllPortsSameDT=off  OutDataTypeStr=boolean
  Logical Operator2 : Logic  Inputs=3  AllPortsSameDT=off  OutDataTypeStr=boolean
  Logical Operator5 : Logic  Operator=OR  Inputs=3  AllPortsSameDT=off  OutDataTypeStr=boolean
  Switch : Switch  Criteria=u2 ~= 0  SaturateOnIntegerOverflow=off  InputSameDT=off
  Terminator4 : Terminator
  TurnOffDelay : Subsystem  AncestorBlock=MAN_Library/TurnOffDelay  mask(Turn Off Delay){CycleTime=Cycle Time: 10 Ms}
      mask prompts: CycleTime "Select the Cycle Time:"
      mask help:
      | This is an EDGE DELAY where the turning-off edge is delayed. The delay period is entered at input PT. The output Q is reset after turning off input IN, only after the delay period is over. Output ET counts the time - beginning with the occurrence of the negative edge - until the value set at PT has been reached. The output ET shows the expired time since turning input IN off until the input state of IN is put through to output Q.
      |
      | IN : Timer starting bit
      | PT : Preset time of timer
      | Q  : Time pulse flag
      | ET : Current value of timer
      mask TypeOptions CycleTime: Cycle Time: 1 Ms | Cycle Time: 10 Ms | Cycle Time: 100 Ms | Cycle Time: 1000 Ms
      mask Display:
      | disp('{\bf\fontsize{18}Turn Off Delay}', 'texmode','on');
      | 
      | port_label('input', 1,'IN');
      | port_label('input', 2,'PT');
      | port_label('output',1,'Q');
      | port_label('output',2,'ET');
  Kitc_StRefgtr : Outport
  "Kitc_StFrntRefgtr " : Outport  Port=2
  wires:
  Data Type Conversion1/1 -> Switch/2
  Constant/1 -> Switch/3
  Data Store Read/1 -> Switch/1, Data Type Conversion1/1
  Logical Operator10/1 -> Kitc_StRefgtr/1
  Toi_ToiInstlldInfo/1 -> Logical Operator10/2
  TurnOffDelay/2(TurnOffDelayExpiredTime) -> Terminator4/1
  Data Type Conversion/1 -> TurnOffDelay/2(TurnOffDelayThreshold)
  Switch/1 -> Data Type Conversion/1
  GW_StClmp15/1 -> Logical Operator9/2, Logical Operator1/1
  Logical Operator9/1 -> "Kitc_StFrntRefgtr "/1
  Logical Operator8/1 -> Logical Operator9/1
  "GW_StUvTopPrio "/1 -> Logical Operator8/1
  Logical Operator7/1 -> Logical Operator6/2
  "GW_StUvLoPrio "/1 -> Logical Operator7/1
  Logical Operator6/1 -> Logical Operator10/1
  TurnOffDelay/1(TurnOffDelayFlag) -> Logical Operator6/1
  Logical Operator5/1 -> TurnOffDelay/1(TurnOffDelayEnable)
  Logical Operator4/1 -> Logical Operator5/3
  Logical Operator1/1 -> Logical Operator5/1
  Logical Operator2/1 -> Logical Operator5/2
  "GW_StEngAcv "/1 -> Logical Operator4/2
  Logical Operator3/1 -> Logical Operator2/3
  Constant3/1 -> Logical Operator3/1, Logical Operator4/1
  GW_StClmpRdo/1 -> Logical Operator2/2
  Logical Operator/1 -> Logical Operator2/1
  Constant2/1 -> Logical Operator/1, Logical Operator1/2

== system Kitchen_Lib/Kitchen/100ms/Kitchn/Subsystem1/Subsystem19/RisingEdgeDetection ==
  CLK : Inport
  Constant : Constant  Value=boolean(1)  OutDataTypeStr=boolean
  Data Type Conversion1 : DataTypeConversion  OutDataTypeStr=boolean  SaturateOnIntegerOverflow=off  RndMeth=Floor
  Logical Operator : Logic  AllPortsSameDT=off  OutDataTypeStr=boolean
  Relational Operator : RelationalOperator  Operator=~=  OutDataTypeStr=boolean  InputSameDT=off
  Relational Operator1 : RelationalOperator  Operator===  OutDataTypeStr=boolean  InputSameDT=off
  Unit Delay : UnitDelay  SampleTime=-1  HasFrameUpgradeWarning=on
  Q : Outport
  wires:
  CLK/1 -> Data Type Conversion1/1
  Unit Delay/1 -> Relational Operator/1
  Relational Operator/1 -> Logical Operator/1
  Relational Operator1/1 -> Logical Operator/2
  Logical Operator/1 -> Q/1
  Constant/1 -> Relational Operator1/2
  Data Type Conversion1/1 -> Unit Delay/1, Relational Operator/2, Relational Operator1/1

== system Kitchen_Lib/Kitchen/100ms/Kitchn/Subsystem1/Subsystem19/SR ==
  S : Inport
  R : Inport  Port=2
  Constant1 : Constant  Value=boolean(1)  OutDataTypeStr=boolean
  Constant3 : Constant  Value=boolean(0)  OutDataTypeStr=boolean
  Data Type Conversion1 : DataTypeConversion  OutDataTypeStr=boolean  SaturateOnIntegerOverflow=off  RndMeth=Floor
  Data Type Conversion2 : DataTypeConversion  OutDataTypeStr=boolean  SaturateOnIntegerOverflow=off  RndMeth=Floor
  Multiport Switch : MultiPortSwitch  DataPortOrder=Zero-based contiguous  Inputs=2  zeroidx=on  SaturateOnIntegerOverflow=off  InputSameDT=off
  Multiport Switch1 : MultiPortSwitch  DataPortOrder=Zero-based contiguous  Inputs=2  zeroidx=on  SaturateOnIntegerOverflow=off  InputSameDT=off
  Unit Delay : UnitDelay  SampleTime=-1  HasFrameUpgradeWarning=on
  Q : Outport
  wires:
  S/1 -> Data Type Conversion2/1
  Constant1/1 -> Multiport Switch/3
  Multiport Switch1/1 -> Multiport Switch/2
  R/1 -> Data Type Conversion1/1
  Unit Delay/1 -> Multiport Switch1/2
  Multiport Switch/1 -> Q/1, Unit Delay/1
  Constant3/1 -> Multiport Switch1/3
  Data Type Conversion1/1 -> Multiport Switch1/1
  Data Type Conversion2/1 -> Multiport Switch/1

== system Kitchen_Lib/Kitchen/100ms/Kitchn/Subsystem1/Subsystem19/TimeConstant ==
  Constant11 : Constant  Value=uint32(hours)  OutDataTypeStr=uint32
  Constant12 : Constant  Value=uint32(minutes)  OutDataTypeStr=uint32
  Constant13 : Constant  Value=uint32(miliseconds)  OutDataTypeStr=uint32
  Constant14 : Constant  Value=uint32(60)  OutDataTypeStr=uint32
  Constant15 : Constant  Value=uint32(1000)  OutDataTypeStr=uint32
  Constant16 : Constant  Value=uint32(seconds)  OutDataTypeStr=uint32
  Constant17 : Constant  Value=uint32(1000)  OutDataTypeStr=uint32
  Constant7 : Constant  Value=uint32(60)  OutDataTypeStr=uint32
  Constant8 : Constant  Value=uint32(60)  OutDataTypeStr=uint32
  Constant9 : Constant  Value=uint32(1000)  OutDataTypeStr=uint32
  Data Type Conversion{1..2,4..8,13..19} (14 alike) : DataTypeConversion  OutDataTypeStr=uint32  SaturateOnIntegerOverflow=off  RndMeth=Floor
  Product1 : Product  Inputs=4  OutDataTypeStr=uint32
  Product2 : Product  Inputs=3  OutDataTypeStr=uint32
  Product4 : Product  OutDataTypeStr=uint32
  Sum1 : Sum  Inputs=++++  AccumDataTypeStr=uint32
  time : Outport
  wires:
  Sum1/1 -> Data Type Conversion5/1  "time"
  Data Type Conversion5/1 -> time/1
  Constant7/1 -> Data Type Conversion13/1
  Data Type Conversion13/1 -> Product1/1
  Constant8/1 -> Data Type Conversion14/1
  Data Type Conversion14/1 -> Product1/2
  Constant9/1 -> Data Type Conversion15/1
  Data Type Conversion15/1 -> Product1/3
  Constant11/1 -> Data Type Conversion16/1
  Data Type Conversion16/1 -> Product1/4
  Constant12/1 -> Data Type Conversion2/1
  Constant14/1 -> Data Type Conversion17/1
  Data Type Conversion17/1 -> Product2/1
  Constant15/1 -> Data Type Conversion18/1
  Data Type Conversion18/1 -> Product2/2
  Constant17/1 -> Data Type Conversion19/1
  Data Type Conversion19/1 -> Product4/1
  Constant16/1 -> Data Type Conversion1/1
  Product1/1 -> Data Type Conversion4/1
  Product2/1 -> Data Type Conversion6/1
  Product4/1 -> Data Type Conversion7/1
  Data Type Conversion1/1 -> Product4/2
  Data Type Conversion2/1 -> Product2/3
  Constant13/1 -> Data Type Conversion8/1
  Data Type Conversion4/1 -> Sum1/1
  Data Type Conversion6/1 -> Sum1/2
  Data Type Conversion7/1 -> Sum1/3
  Data Type Conversion8/1 -> Sum1/4

== system Kitchen_Lib/Kitchen/100ms/Kitchn/Subsystem1/Subsystem19/TimePulse ==
  TimePulseEnable : Inport
  TimePulseDuration : Inport  Port=2
  Constant1 : Constant  Value=uint32(100)  OutDataTypeStr=uint32
  Constant10 : Constant  Value=uint32(CycleTime)  OutDataTypeStr=uint32
  Constant11 : Constant  Value=uint32(1)  OutDataTypeStr=uint32
  Constant12 : Constant  Value=uint32(10)  OutDataTypeStr=uint32
  Constant13 : Constant  Value=uint32(100)  OutDataTypeStr=uint32
  Constant14 : Constant  Value=uint32(1000)  OutDataTypeStr=uint32
  Multiport Switch2 : MultiPortSwitch  Inputs=4  SaturateOnIntegerOverflow=off  InputSameDT=off
  Terminator : Terminator
  TimePulseOriginal : Subsystem  AncestorBlock=MAN_Library/BasicLibrary/TimePulseOriginal
  TimePulseFlag : Outport
  TimePulseExpiredTime : Outport  Port=2
  wires:
  TimePulseOriginal/2(TimePulseExpiredTime) -> TimePulseExpiredTime/1
  TimePulseOriginal/1(TimePulseFlag) -> TimePulseFlag/1
  TimePulseEnable/1 -> TimePulseOriginal/1(TimePulseEnable)
  TimePulseDuration/1 -> TimePulseOriginal/2(TimePulseDuration)
  Constant11/1 -> Multiport Switch2/2
  Constant12/1 -> Multiport Switch2/3
  Constant14/1 -> Multiport Switch2/5
  Constant13/1 -> Multiport Switch2/4
  Constant10/1 -> Multiport Switch2/1
  Multiport Switch2/1 -> Terminator/1
  Constant1/1 -> TimePulseOriginal/3(CycleTime)
